simulink model "sim_test"  (R2020b)
settings: Solver=ode4  StartTime=0.0  StopTime=inf  FixedStep=sim_time  MinStep=0.05/20  RelTol=1e-3
values from neighbouring files (symbols this model uses):
  alpha = 0.127    [main.m]
  cf_max = 2*sqrt(kf*mf)    [main.m]
  cf_min = cf_max/40    [main.m]
  Cl = 2    [main.m]
  cr = 2*sqrt(kr*mr)    [main.m]    (also in state_function.m)
  d_air = 1.18    [main.m]
  elevator_max = 0.5    [main.m]
  Flap_max = 300    [main.m]
  Flap_min = 100    [main.m]
  g = 9.81    [main.m]    (also in state_function.m)
  Jy = (mf*Lf^2)/3    (= 312915.96)    [main.m]    (also in state_function.m)
  Kd_eq = 3    [main.m]
  Kd_lift = 100    [main.m]
  kf = 1e6    (= 1000000)    [main.m]    (also in state_function.m)
  Ki_eq = 3    [main.m]
  Ki_lift = 10    [main.m]
  Kp_eq = 5    [main.m]
  Kp_lift = 1000    [main.m]
  kr = 1e6    (= 1000000)    [main.m]    (also in state_function.m)
  L = - f - v    [lift_control.m]    (also in main.m = 12.6; state_function.m = 12.6)
  Lf = L*0.90    (= 11.34)    [main.m]    (also in state_function.m)
  Lr = L-Lf    (= 1.26)    [main.m]    (also in state_function.m)
  M = 73000    [main.m]    (also in state_function.m)
  Mbrake = 10e1    (= 100)    [main.m]
  sim_time = 0.05/v0x    (= 0.000714285714286)    [main.m]    (also in state_function.m)
  theta0 = (pi/180)*2    (= 0.0349065850399)    [main.m]
  thetad1 = (pi/180)*0    (= 0)    [main.m]
  thetad2 = (pi/180)*4    (= 0.0698131700798)    [main.m]
  v0x = 70    [main.m]    (also in state_function.m)
  z0 = 50    [main.m]
  zd_dot = -1    [main.m]
  zwf0 = z0+Lf*sin(theta0)-((mtf*g/kf)+L0)    [main.m]
  zwr0 = z0-Lr*sin(theta0)-((mtr*g/kr)+L0)    [main.m]
undefined symbols (not defined in the file or in its folder): thetad
libraries: simulink x4, sharedTrackingLibrary x1
settings Model: Creator=alema  LastModifiedBy=alema
settings SolverCC: ZeroCrossAlgorithm=Adaptive
settings DebuggingCC: IgnoredZcDiagnostic=none  UnderSpecifiedDimensionMsg=warning

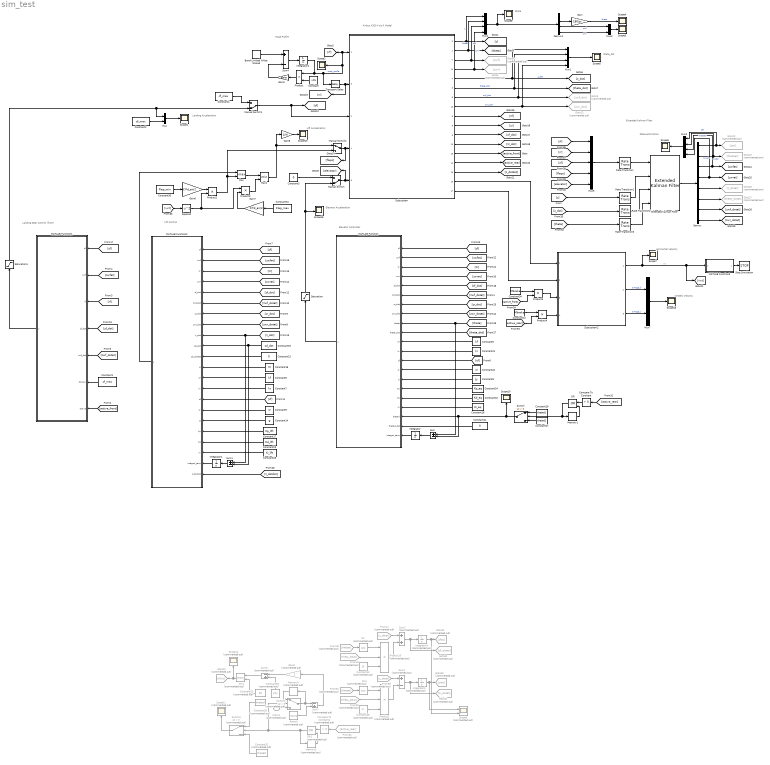
== system sim_test ==
  note: Elevator Controller
  note: Airbus A320 4 d.o.f. Model
  note: Landing Gear Control (front)
  note: Lift Control
  note: Lift Acceleration
  note: Elevator Acceleration
  note: Road Profile
  note: State
  note: Landing Acceleration
  note: State_dot
  note: Extended Kalman Filter
  note: State estimation
  note: Horizontal Velocity
  note: Wheels Velocity
  Band-Limited White Noise3 : simulink/Sources/Band-Limited White Noise  Cov=[2*pi*(4*(4*10^-6))*20*0.127]  Ts=sim_time  seed=[23341]
  Clock1 : Clock  Commented=on
  Compare To Constant : simulink/Logic and Bit Operations/Compare To Constant  relop=>  const=0  OutDataTypeStr=boolean
  Compare To Constant1 : simulink/Logic and Bit Operations/Compare To Constant  Commented=on  relop=>  const=0  OutDataTypeStr=boolean
  Constant : Constant  Value=v0x
  Constant1 : Constant  Value=cf_max
  Constant10 : Constant  Commented=on  Value=Lf
  Constant11 : Constant  Value=0
  Constant12 : Constant  Value=Mbrake
  Constant13 : Constant  Value=0
  Constant14 : Constant  Value=g
  Constant15 : Constant  Value=Kd_eq
  Constant16 : Constant  Value=Ki_eq
  Constant17 : Constant  Value=Kp_lift
  Constant18 : Constant  Value=M
  Constant19 : Constant  Value=zd_dot
  Constant2 : Constant  Value=cf_max
  Constant20 : Constant  Commented=on  Value=20
  Constant21 : Constant  Value=kr
  Constant22 : Constant  Value=cr
  Constant23 : Constant  Value=Kd_lift
  Constant24 : Constant  Value=Kp_eq
  Constant25 : Constant  Value=Ki_lift
  Constant26 : Constant  Value=thetad1
  Constant27 : Constant  Value=thetad2
  Constant28 : Constant  Commented=on  Value=Lr
  Constant29 : Constant  Commented=on  Value=thetad
  Constant3 : Constant  Value=0
  Constant30 : Constant  Value=Flap_min
  Constant31 : Constant  Value=Flap_max
  Constant32 : Constant  Commented=on  Value=theta0
  Constant33 : Constant  Commented=on  Value=v0x
  Constant34 : Constant  Value=Mbrake
  Constant4 : Constant  Value=cf_max
  Constant5 : Constant  Value=kf
  Constant6 : Constant  Value=kf
  Constant7 : Constant  Value=kr
  Constant8 : Constant  Value=Jy
  Constant9 : Constant  Value=cr
  Demux : Demux  Outputs=8
  Demux1 : Demux
  Extended Kalman Filter : sharedTrackingLibrary/Extended Kalman Filter  StateTransitionFcn=state_function  HasStateTransitionJacobianFcn=off  HasAdditiveProcessNoise=Additive  ProcessNoise=1  HasTimeVaryingProcessNoise=off  HasStateTransitionFcnExtraArgument=1  InitialState=[z0,theta0,zwf0,zwr0,0,0,0,0]  InitialStateCovariance=1  MeasurementFcn1=sensor_altimeter  HasMeasurementJacobianFcn1=off  HasMeasurementEnablePort1=off  HasAdditiveMeasurementNoise1=Additive  MeasurementNoise1=1  HasTimeVaryingMeasurementNoise1=off  HasMeasurementFcnExtraArgument1=0  MeasurementFcn2=sensor_vertical_speed  HasMeasurementJacobianFcn2=off  HasMeasurementEnablePort2=off  HasAdditiveMeasurementNoise2=Additive  MeasurementNoise2=1  HasTimeVaryingMeasurementNoise2=off  HasMeasurementFcnExtraArgument2=0  MeasurementFcn3=sensor_attitude  HasMeasurementJacobianFcn3=off  HasMeasurementEnablePort3=off  HasAdditiveMeasurementNoise3=Additive  MeasurementNoise3=1  HasTimeVaryingMeasurementNoise3=off  HasMeasurementFcnExtraArgument3=0  MeasurementFcn4=myMeasurementFcn  HasMeasurementJacobianFcn4=off  HasMeasurementEnablePort4=off  HasAdditiveMeasurementNoise4=Additive  MeasurementNoise4=1  HasTimeVaryingMeasurementNoise4=off  HasMeasurementFcnExtraArgument4=0  MeasurementFcn5=myMeasurementFcn  HasMeasurementJacobianFcn5=off  HasMeasurementEnablePort5=off  HasAdditiveMeasurementNoise5=Additive  MeasurementNoise5=1  HasTimeVaryingMeasurementNoise5=off  HasMeasurementFcnExtraArgument5=0  EnableMultirate=off  StateTransitionFcnSampleTime=1  MeasurementFcn1SampleTime=1  MeasurementFcn2SampleTime=1  MeasurementFcn3SampleTime=1  MeasurementFcn4SampleTime=1  MeasurementFcn5SampleTime=1  UseCurrentEstimator=on  OutputStateCovariance=off  DataType=double  SampleTime=sim_time  NumberOfMeasurements=3
      settings: SourceProductBaseCode=CT,DR,TF,ID,LP,NV,AR,RO,RR,UV,VE
  From34 : From  Commented=on  GotoTag=active_rear
  From47 : From  Commented=on  GotoTag=z_dotat
  From48 : From  Commented=on  GotoTag=thetaat
  From49 : From  Commented=on  GotoTag=theta_dotat
  From50 : From  Commented=on  GotoTag=z_dotat
  From51 : From  Commented=on  GotoTag=thetaat
  From52 : From  Commented=on  GotoTag=theta_dotat
  Gain : Gain  Gain=180/pi
  Gain2 : Gain  Gain=alpha
  Gain3 : Gain  Commented=on
  Gain6 : Gain  Gain=Cl*d_air/2
  Gain7 : Gain  Gain=Cl*d_air/2
  Gain8 : Gain  Gain=1/M
  Goto13 : Goto  Commented=on  GotoTag=zwr_dot
  Goto20 : Goto  Commented=on  GotoTag=v0xt
  Goto22 : Goto  Commented=on  GotoTag=zat
  Goto23 : Goto  Commented=on  GotoTag=thetaat
  Goto26 : Goto  Commented=on  GotoTag=z_dotat
  Goto27 : Goto  Commented=on  GotoTag=theta_dotat
  Goto30 : Goto  Commented=on  GotoTag=zf_dotat
  Goto31 : Goto  Commented=on  GotoTag=zfat
  Goto32 : Goto  Commented=on  GotoTag=zr_dotat
  Goto33 : Goto  Commented=on  GotoTag=zrat
  Goto4 : Goto  Commented=on  GotoTag=zwf
  Goto5 : Goto  Commented=on  GotoTag=zwr
  Goto8 : Goto  Commented=on  GotoTag=zwf_dot
  Integrator : Integrator
  Integrator1 : Integrator
  Integrator2 : Integrator
  Integrator3 : Integrator  Commented=on  InitialCondition=z0+Lf*sin(theta0)
  Integrator4 : Integrator  Commented=on  InitialCondition=z0+Lf*sin(theta0)
  MATLAB Function : MATLAB Function  TreatAsAtomicUnit=on
  MATLAB Function1 : MATLAB Function  TreatAsAtomicUnit=on
  MATLAB Function2 : MATLAB Function  TreatAsAtomicUnit=on
  MATLAB Function3 : MATLAB Function  TreatAsAtomicUnit=on
  Manual Switch : ManualSwitch  CurrentSetting=0
  Manual Switch1 : ManualSwitch  CurrentSetting=0
  Manual Switch2 : ManualSwitch
  Max : MinMax  Function=max  Inputs=2
  Max1 : MinMax  Inputs=2
  Memory1 : Memory
  Memory3 : Memory  Commented=on
  Memory4 : Memory  Commented=on
  Min1 : MinMax  Commented=on  Function=max  Inputs=2
  Mux : Mux  Inputs=2
  Mux1 : Mux
  Mux2 : Mux
  Mux3 : Mux  Inputs=2
  Mux4 : Mux
  Mux5 : Mux  Inputs=5
  Mux7 : Mux  Inputs=2
  OR : Logic  Operator=OR  IconShape=distinctive  AllPortsSameDT=off  OutDataTypeStr=boolean
  OR1 : Logic  Commented=on  Operator=OR  IconShape=distinctive  AllPortsSameDT=off  OutDataTypeStr=boolean
  Product{,2..5} (5 alike) : Product
  Product1 : Product  Commented=on  Inputs=3
  Product15 : Product  Commented=on  Inputs=3
  Ramp1 : simulink/Sources/Ramp  Commented=on  slope=1  start=0  InitialOutput=0
  Rate Transition{,1..3} (4 alike) : RateTransition  OutPortSampleTime=sim_time
  Saturation : Saturate  UpperLimit=elevator_max  LowerLimit=-elevator_max
  Saturation1 : Saturate  UpperLimit=cf_max  LowerLimit=cf_min
  Scope{1..8,10,13,15..16} (12 alike) : Scope
  Scope11 : Scope  Commented=on
  Scope14 : Scope  Commented=on
  Scope9 : Scope  Commented=on  NumInputPorts=2
  Sin : Trigonometry  Commented=on  Operator=cos
  Sin1 : Trigonometry  Commented=on  Operator=cos
  Square2 : Math  Operator=square  SaturateOnIntegerOverflow=on
  Stop Simulation : Stop
  Subsystem : Subsystem  ReferencedSubsystem=model_2dof_gravity
      settings: PortSchema="{\"entries\":[{\"content\":{\"sides\":[{\"content\":{\"connectorIds\":[\"In1\",\"In3\",\"In2\",\"In4\",\"In5\"]},\"type\":\"ConnectorPlacement.EquallySpacedRectSide\",\"uuid\":\"e1757e7e-fa32-484c-bffa-a82ec14c6541\"},{\"content\":{\"connectorIds\":[\"Out2\",\"Out1\",\"Out7\",\"Out11\",\"Out4\",\"Out3\",\"Out8\",\"Out12\",\"Out5\",\"Out9\",\"Out6\",\"Out10\",\"Out13\",\"Out14\",\"Out15\",\"Out16\",\"Out17\"],\"side\":\"RIGHT\"},\"type\":\"ConnectorPlacement.EquallySpacedRectSide\",\"uuid\":\"7023b668-9b1e-4ba3-a016-ebf3779a47a6\"},{\"content\":{\"connectorIds\":[],\"side\":\"TOP\"},\"type\":\"ConnectorPlacement.EquallySpacedRectSide\",\"uuid\":\"68aa4fe4-a135-4fd7-ab63-0a0e25815595\"},{\"content\":{\"connectorIds\":[],\"side\":\"HIDDEN\"},\"type\":\"ConnectorPlacement.EquallySpacedRectSide\",\"uuid\":\"22f9be38-8261-4729-9399-a216241be37f\"}]},\"type\":\"ConnectorPlacement.EquallySpacedConnector\",\"uuid\":\"b87fbbfa-ec79-4017-94e1-64aedc4dc3c8\"}],\"packageUris\":[\"http://schema.mathworks.com/mf0/Connector/R2020b\"],\"version\":\"1.0\"}"
  Subsystem2 : Subsystem  VariantControl=Choice  ReferencedSubsystem=pacejka
  Sum : Sum  Inputs=+-
  Sum1 : Sum  Inputs=+-
  Sum2 : Sum  Commented=on
  Sum3 : Sum  Commented=on  Inputs=+-
  Sum4 : Sum  Inputs=+-
  Sum6 : Sum  Commented=on  Inputs=-+
  Sum7 : Sum  Commented=on  Inputs=-+
  Switch : Switch  Criteria=u2 > Threshold
  Switch1 : Switch  Commented=on  Criteria=u2 > Threshold
  Switch2 : Switch  Commented=on  Criteria=u2 > Threshold
  Transport Delay : TransportDelay  DelayTime=L/20
  wires:
  Band-Limited White Noise3/1 -> Sum4/1
  Sum4/1 -> Integrator2/1
  Subsystem/2 -> Mux4/1, [z]  "z"
  Subsystem/1 -> Mux4/2, [theta]  "theta"
  Subsystem/7 -> Mux4/3, Goto4/1  "zwf"
  Subsystem/11 -> Mux4/4, Goto5/1  "zwr"
  Subsystem/8 -> Mux1/3, Goto8/1  "zwf_dot"
  Subsystem/3 -> [theta_dot], Mux1/2  "theta_dot"
  Subsystem/12 -> Mux1/4, Goto13/1  "zwr_dot"
  Switch/1 -> Sum/2, MATLAB Function/19(thetad), Scope10/1
  MATLAB Function1/1(u) -> Saturation1/1
  Constant1/1 -> MATLAB Function1/6(cf_max)
  [rf] -> MATLAB Function1/3(rf)
  [cf] -> MATLAB Function/13(cf)
  [active_front] -> MATLAB Function1/7(active)
  Subsystem/13 -> [active_front]
  Saturation1/1 -> Manual Switch1/2, Mux/1
  Constant2/1 -> Mux/2
  Mux/1 -> Scope1/1
  Manual Switch/1 -> [elevator], Subsystem/5
  Constant3/1 -> Manual Switch/1
  Manual Switch1/1 -> Subsystem/2, [cf]
  Constant4/1 -> Manual Switch1/1
  [zf] -> MATLAB Function2/1(zf)
  [zwfat] -> MATLAB Function2/2(zwf)
  [zr] -> MATLAB Function2/3(zr)
  [zwrat] -> MATLAB Function2/4(zwr)
  [zwf_dotat] -> MATLAB Function2/6(zwf_dot)
  [zf_dot] -> MATLAB Function2/5(zf_dot)
  [zwr_dotat] -> MATLAB Function2/8(zwr_dot)
  [zr_dot] -> MATLAB Function2/7(zr_dot)
  [cf] -> MATLAB Function2/15(cf)
  Constant9/1 -> MATLAB Function2/16(cr)
  Constant7/1 -> MATLAB Function2/14(kr)
  Constant6/1 -> MATLAB Function2/13(kf)
  Constant14/1 -> MATLAB Function2/17(g)
  Constant17/1 -> MATLAB Function2/18(Kp)
  Constant18/1 -> MATLAB Function2/12(M)
  Constant19/1 -> Sum1/2, MATLAB Function2/10(zd_dot)
  [z_dot] -> Sum1/1, MATLAB Function2/9(z_dot)
  [zf] -> MATLAB Function1/1(zf)
  [zwfat] -> MATLAB Function1/2(zwf)
  [zwf_dotat] -> MATLAB Function1/5(zwf_dot)
  [zf_dot] -> MATLAB Function1/4(zf_dot)
  Subsystem/14 -> [active_rear]
  Subsystem/5 -> [zf]
  Subsystem/9 -> [zr]
  Subsystem/6 -> [zf_dot]
  Subsystem/10 -> [zr_dot]
  Saturation/1 -> Scope15/1, Manual Switch/2
  MATLAB Function/1(u) -> Saturation/1
  Constant5/1 -> MATLAB Function/11(kf)
  Constant21/1 -> MATLAB Function/12(kr)
  Constant22/1 -> MATLAB Function/14(cr)
  Constant24/1 -> MATLAB Function/16(Kp)
  Constant8/1 -> MATLAB Function/15(Jy)
  [zf] -> MATLAB Function/1(zf)
  [zwfat] -> MATLAB Function/2(zwf)
  [zr] -> MATLAB Function/3(zr)
  [zwrat] -> MATLAB Function/4(zwr)
  [zf_dot] -> MATLAB Function/5(zf_dot)
  [zwf_dotat] -> MATLAB Function/6(zwf_dot)
  [zr_dot] -> MATLAB Function/7(zr_dot)
  [zwr_dotat] -> MATLAB Function/8(zwr_dot)
  [theta] -> Sum/1, MATLAB Function/9(theta)
  [theta_dot] -> MATLAB Function/10(theta_dot)
  Constant11/1 -> MATLAB Function/20(thetad_dot)
  Integrator/1 -> MATLAB Function/21(integral_term)
  Sum/1 -> Integrator/1
  Constant15/1 -> MATLAB Function/17(Kd)
  Constant16/1 -> MATLAB Function/18(Ki)
  Integrator1/1 -> MATLAB Function2/21(integral_term)
  Sum1/1 -> Integrator1/1
  Constant13/1 -> MATLAB Function2/11(zd_dotdot)
  Constant23/1 -> MATLAB Function2/19(Kd)
  Constant25/1 -> MATLAB Function2/20(Ki)
  Subsystem/15 -> [z_dotdot]
  [z_dotdot] -> MATLAB Function2/22(z_dotdot)
  Product/1 -> Gain2/1
  Gain2/1 -> Sum4/2
  Constant27/1 -> Switch/3
  [active_rear] -> Compare To Constant/1
  Compare To Constant/1 -> OR/1
  Memory1/1 -> OR/2
  Integrator2/1 -> Scope2/1, Subsystem/1, [rf], Transport Delay/1, Product/1  "road_profle"
  Constant30/1 -> Gain6/1
  Square2/1 -> Product3/1, Product2/2
  [vxt] -> Square2/1
  Gain6/1 -> Product2/1
  Product2/1 -> Manual Switch2/2, Max/2
  Max/1 -> Max1/1
  Constant31/1 -> Gain7/1
  Gain7/1 -> Product3/2
  Product3/1 -> Max1/2
  Max1/1 -> Manual Switch2/1, Gain8/1
  MATLAB Function2/1(L) -> Max/1
  Gain8/1 -> Scope13/1
  Manual Switch2/1 -> [flaps], Subsystem/4
  OR/1 -> Switch/2, Memory1/1
  Constant26/1 -> Switch/1
  Transport Delay/1 -> [rr], Subsystem/3
  Mux4/1 -> Scope8/1, Demux1/1
  Subsystem/4 -> Mux1/1, [z_dot]  "z_dot"
  Constant/1 -> Product/2
  Extended Kalman Filter/1 -> Demux/1
  Mux1/1 -> Scope5/1
  [rf] -> Mux5/1
  [rr] -> Mux5/2
  [cf] -> Mux5/3
  [flaps] -> Mux5/4
  [elevator] -> Mux5/5
  Mux5/1 -> Rate Transition/1
  Rate Transition/1 -> Extended Kalman Filter/1
  [z_dot] -> Rate Transition2/1
  [theta] -> Rate Transition3/1
  Rate Transition1/1 -> Extended Kalman Filter/2
  Rate Transition2/1 -> Extended Kalman Filter/3
  Rate Transition3/1 -> Extended Kalman Filter/4
  [z] -> Rate Transition1/1
  Memory4/1 -> Switch2/1
  Constant20/1 -> Min1/2
  OR1/1 -> Switch1/2, Switch2/2, Memory3/1
  Gain3/1 -> Sum6/1
  Sum7/1 -> Gain3/1
  Constant29/1 -> Switch1/1
  From34/1 -> Compare To Constant1/1
  Switch2/1 -> Sum7/1, Memory4/1
  Sum6/1 -> Min1/1
  Ramp1/1 -> Sum7/2
  Constant32/1 -> Switch1/3
  Constant33/1 -> Sum6/2
  Compare To Constant1/1 -> OR1/1
  Clock1/1 -> Switch2/3
  Memory3/1 -> OR1/2
  Min1/1 -> Scope14/1, Goto20/1
  Switch1/1 -> Scope11/1
  Subsystem/16 -> Subsystem2/1
  Subsystem/17 -> Subsystem2/2
  MATLAB Function3/1(y) -> Stop Simulation/1
  Demux/1 -> Mux2/1, Goto22/1  "zat"
  Demux/2 -> Mux2/2, Goto23/1  "thetaat"
  Demux/3 -> [zwfat], Mux2/3  "zwfat"
  Demux/4 -> Mux2/4, [zwrat]  "zwrat"
  Demux/5 -> Goto26/1
  Demux/6 -> Goto27/1
  Demux/7 -> [zwf_dotat]
  Demux/8 -> [zwr_dotat]
  Mux2/1 -> Scope6/1
  Demux1/3 -> Mux3/1  "zwf"
  Demux1/4 -> Mux3/2  "zwr"
  Mux3/1 -> Scope3/1
  Demux1/2 -> Gain/1
  Gain/1 -> Scope4/1  "theta"
  Product15/1 -> Sum2/2
  Sum2/1 -> Goto30/1, Integrator4/1
  Integrator4/1 -> Scope9/2, Goto31/1
  From48/1 -> Sin/1
  From49/1 -> Product15/2
  Sin/1 -> Product15/1
  From47/1 -> Sum2/1
  Product1/1 -> Sum3/2
  Sum3/1 -> Goto32/1, Integrator3/1
  Integrator3/1 -> Scope9/1, Goto33/1
  From51/1 -> Sin1/1
  Sin1/1 -> Product1/1
  From50/1 -> Sum3/1
  Constant10/1 -> Product15/3
  Constant28/1 -> Product1/3
  From52/1 -> Product1/2
  Product4/1 -> Subsystem2/4
  Constant12/1 -> Product4/1
  [active_rear] -> Product4/2
  [active_front] -> Product5/2
  Constant34/1 -> Product5/1
  Product5/1 -> Subsystem2/3
  Mux7/1 -> Scope16/1
  Subsystem2/1 -> Scope7/1, [vxt], MATLAB Function3/1(u)  "vx"
  Subsystem2/2 -> Mux7/1  "omega_f"
  Subsystem2/3 -> Mux7/2  "omega_r"

== matlab function sim_test/MATLAB Function3 ==
  data: u input; y output
function y = end_simulation(u)
    if u<=0
        y=1;
    else
        y=0;
    end
end

== matlab function sim_test/MATLAB Function1 ==
  data: zf input; zwf input; rf input; zf_dot input; zwf_dot input; u output; cf_max input; active input
function u = function_variational_control_algorithm(zf,zwf,rf,zf_dot,zwf_dot,cf_max,active)

    if active==1
        u=variational_control_algorithm(zf,zwf,rf,zf_dot,zwf_dot);
    else
        u=cf_max;
    end

end

== matlab function sim_test/MATLAB Function ==
  data: zf input; zwf input; zr input; zwr input; u output; zf_dot input; zwf_dot input; zr_dot input; zwr_dot input; theta input; theta_dot input; kf input; kr input; cf input; cr input; Jy input; Kp input; Kd input; Ki input; thetad input; thetad_dot input; integral_term input
function u = function_elevator_control(zf,zwf,zr,zwr,zf_dot,zwf_dot,zr_dot,zwr_dot,theta,theta_dot,kf,kr,cf,cr,Jy,Kp,Kd,Ki,thetad,thetad_dot,integral_term)
    u=elevator_control(zf,zwf,zr,zwr,zf_dot,zwf_dot,zr_dot,zwr_dot,theta,theta_dot,kf,kr,cf,cr,Jy,Kp,Kd,Ki,thetad,thetad_dot,integral_term);
end

== matlab function sim_test/MATLAB Function2 ==
  data: zf input; zwf input; zr input; zwr input; zf_dot input; zwf_dot input; zr_dot input; L output; zwr_dot input; z_dot input; zd_dot input; zd_dotdot input; M input; kf input; kr input; cf input; cr input; g input; Kp input; Kd input; Ki input; integral_term input; z_dotdot input
function L = function_lift_control(zf,zwf,zr,zwr,zf_dot,zwf_dot,zr_dot,zwr_dot,z_dot,zd_dot,zd_dotdot,M,kf,kr,cf,cr,g,Kp,Kd,Ki,integral_term,z_dotdot)  

        L=lift_control(zf,zwf,zr,zwr,zf_dot,zwf_dot,zr_dot,zwr_dot,z_dot,zd_dot,zd_dotdot,M,kf,kr,cf,cr,g,Kp,Kd,Ki,integral_term,z_dotdot);

end
